simulink model "Observer_Controller_Sensors_P3"  (R2022a)
settings: Solver=ode45  StartTime=0.0  StopTime=20  RelTol=1e-3
values from neighbouring files (symbols this model uses):
  A = [0 0 1 0 0 ... (first row only)    [DesignProjectP2.m]    (also in DesignProjectP3.m; DesignProject_OffsetP3.m; mpc_example_regulation.m = [ 	 0,       0,              1,  0, 0; 	 0,       0,        ; mpc_example_tracking.m = [ 	 0,       0,              1,  0, 0; 	 0,       0,        )
  absolute_encoder_counts_per_revolution = 128    [ELEN90064_Project_Parameters.m]
  B = [0;0;0;0;1/La]    [DesignProjectP2.m]    (also in DesignProjectP3.m; DesignProject_OffsetP3.m; mpc_example_regulation.m = [0; 0; 0; 0; 1/La]; mpc_example_tracking.m = [0; 0; 0; 0; 1/La])
  C = [0 1 0 0 0]    [DesignProjectP2.m]    (also in DesignProjectP3.m = [1 0 0 0 0; DesignProject_OffsetP3.m = [1 0 0 0 0; mpc_example_regulation.m = [1 0 0 0 0; mpc_example_tracking.m = [1 0 0 0 0)
  Dp = c2d(Gp, T, 'zoh')    [DesignProjectP3.m]    (also in DesignProject_OffsetP3.m; mpc_example_regulation.m; mpc_example_tracking.m)
  gyro_sigma_drift = deg2rad(5)    [ELEN90064_Project_Parameters.m]
  init = [theta_m_init; theta_l_init; thetadot_m_init; thetadot_l_init; Ia_init]    [ELEN90064_Project_Parameters.m]
  K = K(2:6)    [DesignProjectP2.m]    (also in DesignProjectP3.m = Kr(2:6); DesignProject_OffsetP3.m = K_dist(2:6); phase2_emc.m = place(A,B,desired_poles))
  K_disc = Kr_disc(2:6)    [DesignProjectP3.m]    (also in DesignProject_OffsetP3.m)
  Ki = K(1:2)    [DesignProjectP2.m]    (also in DesignProjectP3.m = Kr(1); DesignProject_OffsetP3.m = K_dist(1))
  Ki_disc = Kr_disc(1)    [DesignProjectP3.m]    (also in DesignProject_OffsetP3.m)
  L = L_t'    [DesignProjectP3.m]    (also in DesignProject_OffsetP3.m; phase2_emc.m = place(A',C',desired_obsv_poles)')
  L_disc = L_disct'    [DesignProjectP3.m]    (also in DesignProject_OffsetP3.m; mpc_example_regulation.m; mpc_example_tracking.m)
  T = 1/50    (= 0.02)    [DesignProjectP3.m]    (also in DesignProject_OffsetP3.m; mpc_example_regulation.m; mpc_example_tracking.m)
  theta_l_init = deg2rad(0)    [ELEN90064_Project_Parameters.m]    (also in mpc_example_regulation.m; mpc_example_tracking.m)
  vision_fps = 50    [ELEN90064_Project_Parameters.m]
settings Model: Creator=Admin  LastModifiedBy=Admin

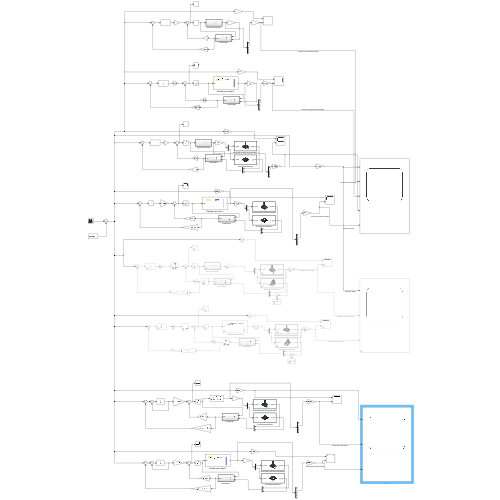
[thumbnail: Simulink's stored preview of the top-level diagram]
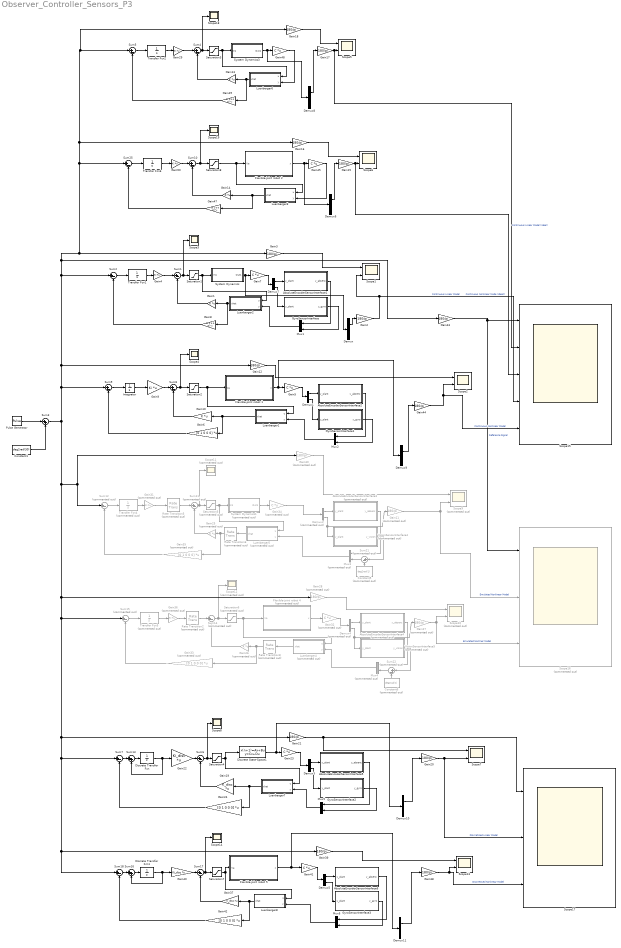
== system Observer_Controller_Sensors_P3 ==
  AbsoluteEncoderSensorInterface1 : Subsystem  TreatAsAtomicUnit=on
      mask Display: image('$imagefile'); % Use "Edit Image" on toolstrip to change.
  AbsoluteEncoderSensorInterface2 : Subsystem  TreatAsAtomicUnit=on
      mask Display: image('$imagefile'); % Use "Edit Image" on toolstrip to change.
  AbsoluteEncoderSensorInterface3 : Subsystem  Commented=on  TreatAsAtomicUnit=on
      mask Display: image('$imagefile'); % Use "Edit Image" on toolstrip to change.
  AbsoluteEncoderSensorInterface4 : Subsystem  Commented=on  TreatAsAtomicUnit=on
      mask Display: image('$imagefile'); % Use "Edit Image" on toolstrip to change.
  AbsoluteEncoderSensorInterface5 : Subsystem  TreatAsAtomicUnit=on
      mask Display: image('$imagefile'); % Use "Edit Image" on toolstrip to change.
  AbsoluteEncoderSensorInterface6 : Subsystem  TreatAsAtomicUnit=on
      mask Display: image('$imagefile'); % Use "Edit Image" on toolstrip to change.
  Constant1 : Constant  Value=deg2rad(30)
  Constant5 : Constant  Commented=on  Value=deg2rad(1)
  Constant6 : Constant  Commented=on  Value=deg2rad(1)
  Demux{,6,8..11} (6 alike) : Demux  Outputs=5
  Demux{1,3,5,7} (4 alike) : Demux  Outputs=2
  Demux2 : Demux  Commented=on  Outputs=2
  Demux4 : Demux  Commented=on  Outputs=2
  Discrete Transfer Fcn : DiscreteTransferFcn  Denominator=[1 0]
  Discrete Transfer Fcn1 : DiscreteTransferFcn  Denominator=[1 0]
  Discrete State-Space1 : DiscreteStateSpace  A=Dp.a  B=Dp.b  C=Dp.c  D=Dp.d  SampleTime=T
  Flexible-joint robot 1 : Subsystem
      mask Display: image('$imagefile'); % Use "Edit Image" on toolstrip to change.
  Flexible-joint robot 2 : Subsystem
      mask Display: image('$imagefile'); % Use "Edit Image" on toolstrip to change.
  Flexible-joint robot 4 : Subsystem  Commented=on
      mask Display: image('$imagefile'); % Use "Edit Image" on toolstrip to change.
  Flexible-joint robot 5 : Subsystem
      mask Display: image('$imagefile'); % Use "Edit Image" on toolstrip to change.
  Gain{1,10,13..14} (4 alike) : Gain  Gain=K  Multiplication=Matrix(K*u)
  Gain{11,27..28,30} (4 alike) : Gain  Commented=on  Gain=180/pi
  Gain{2..3,12,15..18,20..21,38..39,43..44} (13 alike) : Gain  Gain=180/pi
  Gain19 : Gain  Gain=K_disc  Multiplication=Matrix(K*u)
  Gain22 : Gain  Gain=Ki_disc  Multiplication=Matrix(K*u) (u vector)
  Gain{7,23,41,45,48} (5 alike) : Gain  Gain=C  Multiplication=Matrix(K*u)
  Gain{6,8,24,42,47,49} (6 alike) : Gain  Gain=[0 1 0 0 0]  Multiplication=Matrix(K*u)
  Gain25 : Gain  Commented=on  Gain=K  Multiplication=Matrix(K*u)
  Gain26 : Gain  Commented=on  Gain=K  Multiplication=Matrix(K*u)
  Gain29 : Gain  Gain=Ki  Multiplication=Matrix(K*u)
  Gain31 : Gain  Commented=on  Gain=Ki  Multiplication=Matrix(K*u)
  Gain32 : Gain  Commented=on  Gain=C  Multiplication=Matrix(K*u)
  Gain33 : Gain  Commented=on  Gain=[0 1 0 0 0]  Multiplication=Matrix(K*u)
  Gain34 : Gain  Commented=on  Gain=C  Multiplication=Matrix(K*u)
  Gain35 : Gain  Commented=on  Gain=[0 1 0 0 0]  Multiplication=Matrix(K*u)
  Gain36 : Gain  Commented=on  Gain=Ki  Multiplication=Matrix(K*u)
  Gain37 : Gain  Gain=K_disc  Multiplication=Matrix(K*u)
  Gain4 : Gain  Gain=Ki  Multiplication=Matrix(K*u)
  Gain40 : Gain  Gain=Ki_disc  Multiplication=Matrix(K*u)
  Gain5 : Gain  Gain=C  Multiplication=Matrix(K*u) (u vector)
  Gain50 : Gain  Gain=Ki  Multiplication=Matrix(K*u)
  Gain9 : Gain  Gain=Ki  Multiplication=Matrix(K*u) (u vector)
  GyroSensorInterface : Subsystem  TreatAsAtomicUnit=on
      mask Display: image('$imagefile'); % Use "Edit Image" on toolstrip to change.
  GyroSensorInterface1 : Subsystem  TreatAsAtomicUnit=on
      mask Display: image('$imagefile'); % Use "Edit Image" on toolstrip to change.
  GyroSensorInterface2 : Subsystem  TreatAsAtomicUnit=on
      mask Display: image('$imagefile'); % Use "Edit Image" on toolstrip to change.
  GyroSensorInterface3 : Subsystem  TreatAsAtomicUnit=on
      mask Display: image('$imagefile'); % Use "Edit Image" on toolstrip to change.
  Integrator : Integrator
  Luenberger1 : Subsystem  TreatAsAtomicUnit=on
  Luenberger2 : Subsystem  TreatAsAtomicUnit=on
  Luenberger3 : Subsystem  TreatAsAtomicUnit=on
  Luenberger4 : Subsystem  Commented=on  TreatAsAtomicUnit=on
  Luenberger5 : Subsystem  Commented=on  TreatAsAtomicUnit=on
  Luenberger6 : Subsystem  TreatAsAtomicUnit=on
  Luenberger7 : Subsystem  TreatAsAtomicUnit=on
  Luenberger8 : Subsystem  TreatAsAtomicUnit=on
  Mux{1..2,5..6} (4 alike) : Mux  Inputs=2
  Mux3 : Mux  Commented=on  Inputs=2
  Mux4 : Mux  Commented=on  Inputs=2
  Pulse Generator : DiscretePulseGenerator  PulseType=Time based  Amplitude=deg2rad(30)  Period=5  PulseWidth=50
  Rate Transition{2,5..6,8} (4 alike) : RateTransition  Commented=on  OutPortSampleTime=T
  Saturation{1..4,7..8} (6 alike) : Saturate  UpperLimit=6  LowerLimit=-6
  Saturation5 : Saturate  Commented=on  UpperLimit=6  LowerLimit=-6
  Saturation6 : Saturate  Commented=on  UpperLimit=6  LowerLimit=-6
  Scope{1..2,5..7,13} (6 alike) : Scope  NumInputPorts=2
  Scope10 : Scope  Commented=on  NumInputPorts=2
  Scope11 : Scope  Commented=on
  Scope12 : Scope  Commented=on
  Scope{3..4,8,14,18..19} (6 alike) : Scope
  Scope15 : Scope  NumInputPorts=5
  Scope16 : Scope  Commented=on  NumInputPorts=3
  Scope17 : Scope  NumInputPorts=3
  Scope9 : Scope  Commented=on  NumInputPorts=2
  Sum{1..2,4..10,17..18,25} (12 alike) : Sum  Inputs=|+-
  Sum{11..12,14..15,21..22} (6 alike) : Sum  Commented=on  Inputs=|+-
  Sum13 : Sum  Inputs=|++
  Sum16 : Sum  Inputs=|++
  Sum3 : Sum  Inputs=|++
  System Dynamics : Subsystem  TreatAsAtomicUnit=on
  System Dynamics1 : Subsystem  Commented=on  TreatAsAtomicUnit=on
  System Dynamics3 : Subsystem  TreatAsAtomicUnit=on
  Transfer Fcn1 : TransferFcn  Denominator=[1 0]
  Transfer Fcn2 : TransferFcn  Denominator=[1 0]
  Transfer Fcn4 : TransferFcn  Commented=on  Denominator=[1 0]
  Transfer Fcn5 : TransferFcn  Commented=on  Denominator=[1 0]
  Transfer Fcn6 : TransferFcn  Denominator=[1 0]
  VisionSensorInterface4 : Subsystem  Commented=on  TreatAsAtomicUnit=on
      mask Display: image('$imagefile'); % Use "Edit Image" on toolstrip to change.
  VisionSensorInterface5 : Subsystem  Commented=on  TreatAsAtomicUnit=on
      mask Display: image('$imagefile'); % Use "Edit Image" on toolstrip to change.
  wires:
  Sum8/1 -> Scope4/1, Saturation2/1
  Saturation2/1 -> Luenberger1/1(u), Flexible-joint robot 1/1(Va)
  Sum9/1 -> Integrator/1
  Gain10/1 -> Sum8/2
  Integrator/1 -> Gain9/1
  Flexible-joint robot 1/1(x) -> Demux9/1, Gain5/1
  Gain12/1 -> Scope2/1
  Gain44/1 -> Scope2/2, Scope15/5  "Continuous Nonlinear Model"
  Luenberger1/1(xhat) -> Gain6/1, Gain10/1
  Gain6/1 -> Sum9/2
  Gain9/1 -> Sum8/1
  Gain2/1 -> Scope1/2, Scope15/4  "Continuous Linear Model"
  Gain3/1 -> Scope1/1
  Transfer Fcn1/1 -> Gain4/1
  Gain1/1 -> Sum1/2
  Sum2/1 -> Transfer Fcn1/1
  Sum1/1 -> Scope3/1, Saturation1/1
  Gain8/1 -> Sum2/2
  Gain4/1 -> Sum1/1
  Saturation1/1 -> Luenberger2/1(u), System Dynamics/1(In1)
  Luenberger2/1(xhat) -> Gain8/1, Gain1/1
  Pulse Generator/1 -> Sum3/1
  System Dynamics/1(Out1) -> Demux/1, Gain7/1
  Constant1/1 -> Sum3/2
  Luenberger7/1(xhat) -> Gain24/1, Gain19/1
  Saturation4/1 -> Luenberger7/1(u), Discrete State-Space1/1
  Gain22/1 -> Sum6/1
  Gain24/1 -> Sum7/2
  Sum6/1 -> Saturation4/1, Scope8/1
  Gain19/1 -> Sum6/2
  Gain21/1 -> Scope17/1, Scope7/1
  Gain20/1 -> Scope17/2, Scope7/2  "Discretised Linear Model"
  Sum13/1 -> Discrete Transfer Fcn/1
  Discrete Transfer Fcn/1 -> Gain22/1, Sum13/2
  Sum7/1 -> Sum13/1
  Gain23/1 -> Demux3/1
  System Dynamics1/1(Out1) -> Gain34/1
  Luenberger5/1(xhat) -> Rate Transition6/1
  Saturation5/1 -> System Dynamics1/1(In1), Luenberger5/1(u)
  Gain31/1 -> Rate Transition5/1
  Gain35/1 -> Sum12/2
  Sum11/1 -> Saturation5/1, Scope11/1
  Sum12/1 -> Transfer Fcn4/1
  Gain25/1 -> Sum11/2
  Transfer Fcn4/1 -> Gain31/1
  Gain30/1 -> Scope9/1
  Gain36/1 -> Rate Transition2/1
  Gain33/1 -> Sum15/2
  Luenberger4/1(xhat) -> Rate Transition8/1
  Gain32/1 -> Demux4/1
  Gain27/1 -> Scope10/2, Scope16/3  "Emulated Nonliner Model"
  Gain28/1 -> Scope10/1
  Flexible-joint robot 4/1(x) -> Gain32/1
  Transfer Fcn5/1 -> Gain36/1
  Sum15/1 -> Transfer Fcn5/1
  Saturation6/1 -> Flexible-joint robot 4/1(Va), Luenberger4/1(u)
  Sum14/1 -> Saturation6/1, Scope12/1
  Gain26/1 -> Sum14/2
  Rate Transition2/1 -> Sum14/1
  Gain41/1 -> Demux5/1
  Sum18/1 -> Sum16/1
  Discrete Transfer Fcn1/1 -> Sum16/2, Gain40/1
  Sum16/1 -> Discrete Transfer Fcn1/1
  Gain38/1 -> Scope13/2, Scope17/3  "Discretised Nonlinear Model"
  Gain39/1 -> Scope13/1
  Gain37/1 -> Sum17/2
  Sum17/1 -> Scope14/1, Saturation7/1
  Gain42/1 -> Sum18/2
  Gain40/1 -> Sum17/1
  Saturation7/1 -> Flexible-joint robot 5/1(Va), Luenberger8/1(u)
  Luenberger8/1(xhat) -> Gain37/1, Gain42/1
  Rate Transition5/1 -> Sum11/1
  Rate Transition6/1 -> Gain35/1, Gain25/1
  Gain43/1 -> Scope16/1, Scope15/1  "Reference Signal"
  Rate Transition8/1 -> Gain33/1, Gain26/1
  GyroSensorInterface/1(y_gyro) -> Mux1/2
  AbsoluteEncoderSensorInterface1/1(y_absenc) -> Mux1/1
  Gain7/1 -> Demux7/1
  Demux7/2 -> GyroSensorInterface/1(y_plant)
  Demux7/1 -> AbsoluteEncoderSensorInterface1/1(y_plant)
  Mux1/1 -> Luenberger2/2(y)
  Mux2/1 -> Luenberger1/2(y)
  Demux1/1 -> AbsoluteEncoderSensorInterface2/1(y_plant)
  Demux1/2 -> GyroSensorInterface1/1(y_plant)
  Gain5/1 -> Demux1/1
  AbsoluteEncoderSensorInterface2/1(y_absenc) -> Mux2/1
  GyroSensorInterface1/1(y_gyro) -> Mux2/2
  VisionSensorInterface4/1(y_vision) -> Sum21/1
  Constant5/1 -> Sum21/2
  Sum21/1 -> Mux3/2
  AbsoluteEncoderSensorInterface3/1(y_absenc) -> Mux3/1
  Demux2/2 -> Gain11/1, VisionSensorInterface4/1(y_plant)
  Demux2/1 -> AbsoluteEncoderSensorInterface3/1(y_plant)
  Mux3/1 -> Luenberger5/2(y)
  Gain34/1 -> Demux2/1
  Gain11/1 -> Scope9/2, Scope16/2  "Emulated Nonlinear Model"
  Mux4/1 -> Luenberger4/2(y)
  Demux4/1 -> AbsoluteEncoderSensorInterface4/1(y_plant)
  Demux4/2 -> VisionSensorInterface5/1(y_plant), Gain27/1
  AbsoluteEncoderSensorInterface4/1(y_absenc) -> Mux4/1
  Sum22/1 -> Mux4/2
  Constant6/1 -> Sum22/2
  VisionSensorInterface5/1(y_vision) -> Sum22/1
  AbsoluteEncoderSensorInterface5/1(y_absenc) -> Mux5/1
  Demux3/1 -> AbsoluteEncoderSensorInterface5/1(y_plant)
  Demux3/2 -> GyroSensorInterface2/1(y_plant)
  Demux5/2 -> GyroSensorInterface3/1(y_plant)
  Demux5/1 -> AbsoluteEncoderSensorInterface6/1(y_plant)
  AbsoluteEncoderSensorInterface6/1(y_absenc) -> Mux6/1
  GyroSensorInterface3/1(y_gyro) -> Mux6/2
  Gain18/1 -> Scope5/1
  Transfer Fcn6/1 -> Gain50/1
  Sum4/1 -> Scope18/1, Saturation3/1
  Sum25/1 -> Transfer Fcn6/1
  Gain48/1 -> Luenberger6/2(y)
  Saturation3/1 -> Luenberger6/1(u), System Dynamics3/1(In1)
  Gain29/1 -> Sum4/1
  Gain14/1 -> Sum10/2
  Transfer Fcn2/1 -> Gain29/1
  Gain17/1 -> Scope15/2, Scope5/2  "Continuous Linear Model (Ideal)"
  System Dynamics3/1(Out1) -> Demux8/1, Gain48/1
  Gain13/1 -> Sum4/2
  Luenberger6/1(xhat) -> Gain49/1, Gain13/1
  Gain49/1 -> Sum5/2
  Gain47/1 -> Sum25/2
  Gain50/1 -> Sum10/1
  Saturation8/1 -> Luenberger3/1(u), Flexible-joint robot 2/1(Va)
  Gain15/1 -> Scope15/3, Scope6/2  "Continuous Nonlinear Mode (Ideal)l"
  Sum10/1 -> Scope19/1, Saturation8/1
  Demux8/2 -> Gain17/1
  Sum5/1 -> Transfer Fcn2/1
  Gain16/1 -> Scope6/1
  Sum3/1 -> Gain12/1, Gain18/1, Sum5/1, Gain16/1, Sum25/1, Gain3/1, Gain43/1, Sum2/1, Sum9/1, Sum12/1, Gain30/1, Gain28/1, Gain21/1, Sum18/1, Gain39/1, Sum7/1, Sum15/1
  Discrete State-Space1/1 -> Demux10/1, Gain23/1
  Flexible-joint robot 5/1(x) -> Demux11/1, Gain41/1
  GyroSensorInterface2/1(y_gyro) -> Mux5/2
  Demux6/2 -> Gain15/1
  Demux/2 -> Gain2/1
  Demux9/2 -> Gain44/1
  Flexible-joint robot 2/1(x) -> Demux6/1, Gain45/1
  Gain45/1 -> Luenberger3/2(y)
  Luenberger3/1(xhat) -> Gain47/1, Gain14/1
  Mux5/1 -> Luenberger7/2(y)
  Demux10/2 -> Gain20/1
  Demux11/2 -> Gain38/1
  Mux6/1 -> Luenberger8/2(y)

== system Observer_Controller_Sensors_P3/AbsoluteEncoderSensorInterface1 ==
  note: Notes:
      | > This sensor block is protected.
      | > The AbsoluteEncoderSensor.slxp file needs to be on the Matlab path in order to simulate this sensor.
      | > You should have download the .slpx file appropriate for you operating system {Windows, Mac, Linux}.
      | > The constant parameters on the left are set in the " ELEN90064_Project_Parameters.m " script.
      | > The sensors appendix in project description provides a 1-page summary of the sensor model and of how each parameters relates to the expected performance of the sensor.
      | > You should read the relevant page of that appendix before using this sensor.
  y_plant : Inport
  AbsoluteEncoderSensor : ModelReference  ModelNameDialog=AbsoluteEncoderSensor.slxp  ModelReferenceVersion=1.16  CopyOfModelProtected=on
  NUMBER OF COUNTS PER REVOLUTION : Constant  Value=absolute_encoder_counts_per_revolution
  y_absenc : Outport
  wires:
  NUMBER OF COUNTS PER REVOLUTION/1 -> AbsoluteEncoderSensor/1
  y_plant/1 -> AbsoluteEncoderSensor/2
  AbsoluteEncoderSensor/1 -> y_absenc/1

== system Observer_Controller_Sensors_P3/AbsoluteEncoderSensorInterface2 ==
  note: Notes:
      | > This sensor block is protected.
      | > The AbsoluteEncoderSensor.slxp file needs to be on the Matlab path in order to simulate this sensor.
      | > You should have download the .slpx file appropriate for you operating system {Windows, Mac, Linux}.
      | > The constant parameters on the left are set in the " ELEN90064_Project_Parameters.m " script.
      | > The sensors appendix in project description provides a 1-page summary of the sensor model and of how each parameters relates to the expected performance of the sensor.
      | > You should read the relevant page of that appendix before using this sensor.
  y_plant : Inport
  AbsoluteEncoderSensor : ModelReference  ModelNameDialog=AbsoluteEncoderSensor.slxp  ModelReferenceVersion=1.16  CopyOfModelProtected=on
  NUMBER OF COUNTS PER REVOLUTION : Constant  Value=absolute_encoder_counts_per_revolution
  y_absenc : Outport
  wires:
  AbsoluteEncoderSensor/1 -> y_absenc/1
  y_plant/1 -> AbsoluteEncoderSensor/2
  NUMBER OF COUNTS PER REVOLUTION/1 -> AbsoluteEncoderSensor/1

== system Observer_Controller_Sensors_P3/AbsoluteEncoderSensorInterface3 ==
  note: Notes:
      | > This sensor block is protected.
      | > The AbsoluteEncoderSensor.slxp file needs to be on the Matlab path in order to simulate this sensor.
      | > You should have download the .slpx file appropriate for you operating system {Windows, Mac, Linux}.
      | > The constant parameters on the left are set in the " ELEN90064_Project_Parameters.m " script.
      | > The sensors appendix in project description provides a 1-page summary of the sensor model and of how each parameters relates to the expected performance of the sensor.
      | > You should read the relevant page of that appendix before using this sensor.
  y_plant : Inport
  AbsoluteEncoderSensor : ModelReference  ModelNameDialog=AbsoluteEncoderSensor.slxp  ModelReferenceVersion=1.16  CopyOfModelProtected=on
  NUMBER OF COUNTS PER REVOLUTION : Constant  Value=absolute_encoder_counts_per_revolution
  y_absenc : Outport
  wires:
  NUMBER OF COUNTS PER REVOLUTION/1 -> AbsoluteEncoderSensor/1
  y_plant/1 -> AbsoluteEncoderSensor/2
  AbsoluteEncoderSensor/1 -> y_absenc/1

== system Observer_Controller_Sensors_P3/AbsoluteEncoderSensorInterface4 ==
  note: Notes:
      | > This sensor block is protected.
      | > The AbsoluteEncoderSensor.slxp file needs to be on the Matlab path in order to simulate this sensor.
      | > You should have download the .slpx file appropriate for you operating system {Windows, Mac, Linux}.
      | > The constant parameters on the left are set in the " ELEN90064_Project_Parameters.m " script.
      | > The sensors appendix in project description provides a 1-page summary of the sensor model and of how each parameters relates to the expected performance of the sensor.
      | > You should read the relevant page of that appendix before using this sensor.
  y_plant : Inport
  AbsoluteEncoderSensor : ModelReference  ModelNameDialog=AbsoluteEncoderSensor.slxp  ModelReferenceVersion=1.16  CopyOfModelProtected=on
  NUMBER OF COUNTS PER REVOLUTION : Constant  Value=absolute_encoder_counts_per_revolution
  y_absenc : Outport
  wires:
  AbsoluteEncoderSensor/1 -> y_absenc/1
  y_plant/1 -> AbsoluteEncoderSensor/2
  NUMBER OF COUNTS PER REVOLUTION/1 -> AbsoluteEncoderSensor/1

== system Observer_Controller_Sensors_P3/AbsoluteEncoderSensorInterface5 ==
  note: Notes:
      | > This sensor block is protected.
      | > The AbsoluteEncoderSensor.slxp file needs to be on the Matlab path in order to simulate this sensor.
      | > You should have download the .slpx file appropriate for you operating system {Windows, Mac, Linux}.
      | > The constant parameters on the left are set in the " ELEN90064_Project_Parameters.m " script.
      | > The sensors appendix in project description provides a 1-page summary of the sensor model and of how each parameters relates to the expected performance of the sensor.
      | > You should read the relevant page of that appendix before using this sensor.
  y_plant : Inport
  AbsoluteEncoderSensor : ModelReference  ModelNameDialog=AbsoluteEncoderSensor.slxp  ModelReferenceVersion=1.16  CopyOfModelProtected=on
  NUMBER OF COUNTS PER REVOLUTION : Constant  Value=absolute_encoder_counts_per_revolution
  y_absenc : Outport
  wires:
  NUMBER OF COUNTS PER REVOLUTION/1 -> AbsoluteEncoderSensor/1
  y_plant/1 -> AbsoluteEncoderSensor/2
  AbsoluteEncoderSensor/1 -> y_absenc/1

== system Observer_Controller_Sensors_P3/AbsoluteEncoderSensorInterface6 ==
  note: Notes:
      | > This sensor block is protected.
      | > The AbsoluteEncoderSensor.slxp file needs to be on the Matlab path in order to simulate this sensor.
      | > You should have download the .slpx file appropriate for you operating system {Windows, Mac, Linux}.
      | > The constant parameters on the left are set in the " ELEN90064_Project_Parameters.m " script.
      | > The sensors appendix in project description provides a 1-page summary of the sensor model and of how each parameters relates to the expected performance of the sensor.
      | > You should read the relevant page of that appendix before using this sensor.
  y_plant : Inport
  AbsoluteEncoderSensor : ModelReference  ModelNameDialog=AbsoluteEncoderSensor.slxp  ModelReferenceVersion=1.16  CopyOfModelProtected=on
  NUMBER OF COUNTS PER REVOLUTION : Constant  Value=absolute_encoder_counts_per_revolution
  y_absenc : Outport
  wires:
  AbsoluteEncoderSensor/1 -> y_absenc/1
  y_plant/1 -> AbsoluteEncoderSensor/2
  NUMBER OF COUNTS PER REVOLUTION/1 -> AbsoluteEncoderSensor/1

== system Observer_Controller_Sensors_P3/Flexible-joint robot 1 ==
  Va : Inport
  Constant : Constant  Value=init
  Constant1 : Constant  Value=0
  Flexible-joint robot 1 : ModelReference  ModelNameDialog=Flexible_joint_robot_1  ModelReferenceVersion=1.65  CopyOfModelProtected=on
  Step : Step  After=0.05  SampleTime=0
  x : Outport
  wires:
  Constant/1 -> Flexible-joint robot 1/2
  Constant1/1 -> Flexible-joint robot 1/3
  Flexible-joint robot 1/1 -> x/1
  Va/1 -> Flexible-joint robot 1/1

== system Observer_Controller_Sensors_P3/Flexible-joint robot 2 ==
  Va : Inport
  Constant : Constant  Value=init
  Constant1 : Constant  Value=0
  Flexible-joint robot 1 : ModelReference  ModelNameDialog=Flexible_joint_robot_1  ModelReferenceVersion=1.65  CopyOfModelProtected=on
  Step : Step  After=0.05  SampleTime=0
  x : Outport
  wires:
  Constant/1 -> Flexible-joint robot 1/2
  Constant1/1 -> Flexible-joint robot 1/3
  Flexible-joint robot 1/1 -> x/1
  Va/1 -> Flexible-joint robot 1/1

== system Observer_Controller_Sensors_P3/Flexible-joint robot 4 ==
  Va : Inport
  Constant : Constant  Value=init
  Constant1 : Constant  Value=0
  Flexible-joint robot 1 : ModelReference  ModelNameDialog=Flexible_joint_robot_1  ModelReferenceVersion=1.65  CopyOfModelProtected=on
  Step : Step  After=0.05  SampleTime=0
  x : Outport
  wires:
  Va/1 -> Flexible-joint robot 1/1
  Flexible-joint robot 1/1 -> x/1
  Constant1/1 -> Flexible-joint robot 1/3
  Constant/1 -> Flexible-joint robot 1/2

== system Observer_Controller_Sensors_P3/Flexible-joint robot 5 ==
  Va : Inport
  Constant : Constant  Value=init
  Constant1 : Constant  Value=0
  Flexible-joint robot 1 : ModelReference  ModelNameDialog=Flexible_joint_robot_1  ModelReferenceVersion=1.65  CopyOfModelProtected=on
  Step : Step  After=0.05  SampleTime=0
  x : Outport
  wires:
  Constant/1 -> Flexible-joint robot 1/2
  Constant1/1 -> Flexible-joint robot 1/3
  Flexible-joint robot 1/1 -> x/1
  Va/1 -> Flexible-joint robot 1/1

== system Observer_Controller_Sensors_P3/GyroSensorInterface ==
  note: Notes:
      | > This sensor block is protected.
      | > The GyroSensor.slxp file needs to be on the Matlab path in order to simulate this sensor.
      | > You should have download the .slpx file appropriate for you operating system {Windows, Mac, Linux}.
      | > The constant parameters on the left are set in the " ELEN90064_Project_Parameters.m " script.
      | > The sensors appendix in project description provides a 1-page summary of the sensor model and of how each parameters relates to the expected performance of the sensor.
      | > You should read the relevant page of that appendix before using this sensor.
  y_plant : Inport
  GYRO SIGMA DRIFT [rad/s^2] : Constant  Value=gyro_sigma_drift
  GyroSensor : ModelReference  ModelNameDialog=GyroSensor.slxp  ModelReferenceVersion=1.18  CopyOfModelProtected=on
  y_gyro : Outport
  wires:
  GYRO SIGMA DRIFT [rad/s^2]/1 -> GyroSensor/1
  y_plant/1 -> GyroSensor/2
  GyroSensor/1 -> y_gyro/1

== system Observer_Controller_Sensors_P3/GyroSensorInterface1 ==
  note: Notes:
      | > This sensor block is protected.
      | > The GyroSensor.slxp file needs to be on the Matlab path in order to simulate this sensor.
      | > You should have download the .slpx file appropriate for you operating system {Windows, Mac, Linux}.
      | > The constant parameters on the left are set in the " ELEN90064_Project_Parameters.m " script.
      | > The sensors appendix in project description provides a 1-page summary of the sensor model and of how each parameters relates to the expected performance of the sensor.
      | > You should read the relevant page of that appendix before using this sensor.
  y_plant : Inport
  GYRO SIGMA DRIFT [rad/s^2] : Constant  Value=gyro_sigma_drift
  GyroSensor : ModelReference  ModelNameDialog=GyroSensor.slxp  ModelReferenceVersion=1.18  CopyOfModelProtected=on
  y_gyro : Outport
  wires:
  GYRO SIGMA DRIFT [rad/s^2]/1 -> GyroSensor/1
  y_plant/1 -> GyroSensor/2
  GyroSensor/1 -> y_gyro/1

== system Observer_Controller_Sensors_P3/GyroSensorInterface2 ==
  note: Notes:
      | > This sensor block is protected.
      | > The GyroSensor.slxp file needs to be on the Matlab path in order to simulate this sensor.
      | > You should have download the .slpx file appropriate for you operating system {Windows, Mac, Linux}.
      | > The constant parameters on the left are set in the " ELEN90064_Project_Parameters.m " script.
      | > The sensors appendix in project description provides a 1-page summary of the sensor model and of how each parameters relates to the expected performance of the sensor.
      | > You should read the relevant page of that appendix before using this sensor.
  y_plant : Inport
  GYRO SIGMA DRIFT [rad/s^2] : Constant  Value=gyro_sigma_drift
  GyroSensor : ModelReference  ModelNameDialog=GyroSensor.slxp  ModelReferenceVersion=1.18  CopyOfModelProtected=on
  y_gyro : Outport
  wires:
  GYRO SIGMA DRIFT [rad/s^2]/1 -> GyroSensor/1
  y_plant/1 -> GyroSensor/2
  GyroSensor/1 -> y_gyro/1

== system Observer_Controller_Sensors_P3/GyroSensorInterface3 ==
  note: Notes:
      | > This sensor block is protected.
      | > The GyroSensor.slxp file needs to be on the Matlab path in order to simulate this sensor.
      | > You should have download the .slpx file appropriate for you operating system {Windows, Mac, Linux}.
      | > The constant parameters on the left are set in the " ELEN90064_Project_Parameters.m " script.
      | > The sensors appendix in project description provides a 1-page summary of the sensor model and of how each parameters relates to the expected performance of the sensor.
      | > You should read the relevant page of that appendix before using this sensor.
  y_plant : Inport
  GYRO SIGMA DRIFT [rad/s^2] : Constant  Value=gyro_sigma_drift
  GyroSensor : ModelReference  ModelNameDialog=GyroSensor.slxp  ModelReferenceVersion=1.18  CopyOfModelProtected=on
  y_gyro : Outport
  wires:
  GYRO SIGMA DRIFT [rad/s^2]/1 -> GyroSensor/1
  y_plant/1 -> GyroSensor/2
  GyroSensor/1 -> y_gyro/1

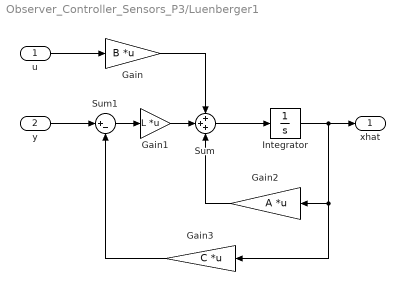
== system Observer_Controller_Sensors_P3/Luenberger1 ==
  u : Inport
  y : Inport  Port=2
  Gain : Gain  Gain=B  Multiplication=Matrix(K*u) (u vector)
  Gain1 : Gain  Gain=L  Multiplication=Matrix(K*u) (u vector)
  Gain2 : Gain  Gain=A  Multiplication=Matrix(K*u) (u vector)
  Gain3 : Gain  Gain=C  Multiplication=Matrix(K*u) (u vector)
  Integrator : Integrator
  Sum : Sum  Inputs=+++
  Sum1 : Sum  Inputs=|+-
  xhat : Outport
  wires:
  u/1 -> Gain/1
  Gain/1 -> Sum/1
  y/1 -> Sum1/1
  Sum1/1 -> Gain1/1
  Gain1/1 -> Sum/2
  Sum/1 -> Integrator/1
  Integrator/1 -> Gain3/1, Gain2/1, xhat/1
  Gain2/1 -> Sum/3
  Gain3/1 -> Sum1/2

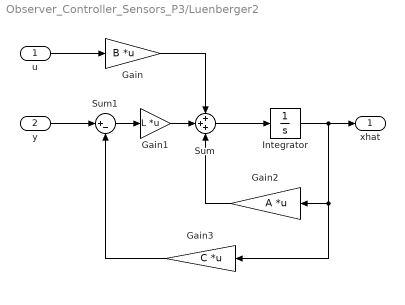
== system Observer_Controller_Sensors_P3/Luenberger2 ==
  u : Inport
  y : Inport  Port=2
  Gain : Gain  Gain=B  Multiplication=Matrix(K*u) (u vector)
  Gain1 : Gain  Gain=L  Multiplication=Matrix(K*u) (u vector)
  Gain2 : Gain  Gain=A  Multiplication=Matrix(K*u) (u vector)
  Gain3 : Gain  Gain=C  Multiplication=Matrix(K*u) (u vector)
  Integrator : Integrator
  Sum : Sum  Inputs=+++
  Sum1 : Sum  Inputs=|+-
  xhat : Outport
  wires:
  u/1 -> Gain/1
  Gain/1 -> Sum/1
  y/1 -> Sum1/1
  Sum1/1 -> Gain1/1
  Gain1/1 -> Sum/2
  Sum/1 -> Integrator/1
  Integrator/1 -> Gain3/1, Gain2/1, xhat/1
  Gain2/1 -> Sum/3
  Gain3/1 -> Sum1/2

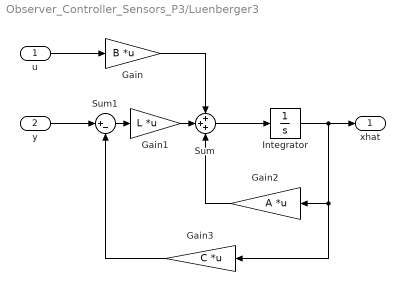
== system Observer_Controller_Sensors_P3/Luenberger3 ==
  u : Inport
  y : Inport  Port=2
  Gain : Gain  Gain=B  Multiplication=Matrix(K*u) (u vector)
  Gain1 : Gain  Gain=L  Multiplication=Matrix(K*u) (u vector)
  Gain2 : Gain  Gain=A  Multiplication=Matrix(K*u) (u vector)
  Gain3 : Gain  Gain=C  Multiplication=Matrix(K*u) (u vector)
  Integrator : Integrator
  Sum : Sum  Inputs=+++
  Sum1 : Sum  Inputs=|+-
  xhat : Outport
  wires:
  u/1 -> Gain/1
  Gain/1 -> Sum/1
  y/1 -> Sum1/1
  Sum1/1 -> Gain1/1
  Gain1/1 -> Sum/2
  Sum/1 -> Integrator/1
  Integrator/1 -> Gain3/1, Gain2/1, xhat/1
  Gain2/1 -> Sum/3
  Gain3/1 -> Sum1/2

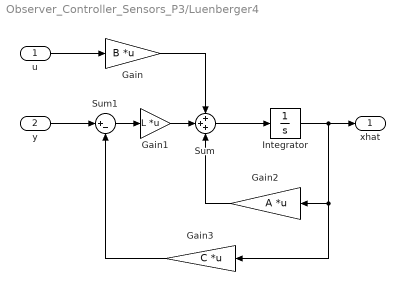
== system Observer_Controller_Sensors_P3/Luenberger4 ==
  u : Inport
  y : Inport  Port=2
  Gain : Gain  Gain=B  Multiplication=Matrix(K*u) (u vector)
  Gain1 : Gain  Gain=L  Multiplication=Matrix(K*u) (u vector)
  Gain2 : Gain  Gain=A  Multiplication=Matrix(K*u) (u vector)
  Gain3 : Gain  Gain=C  Multiplication=Matrix(K*u) (u vector)
  Integrator : Integrator
  Sum : Sum  Inputs=+++
  Sum1 : Sum  Inputs=|+-
  xhat : Outport
  wires:
  Gain3/1 -> Sum1/2
  Gain2/1 -> Sum/3
  Integrator/1 -> xhat/1, Gain2/1, Gain3/1
  Sum/1 -> Integrator/1
  Gain1/1 -> Sum/2
  Sum1/1 -> Gain1/1
  y/1 -> Sum1/1
  Gain/1 -> Sum/1
  u/1 -> Gain/1

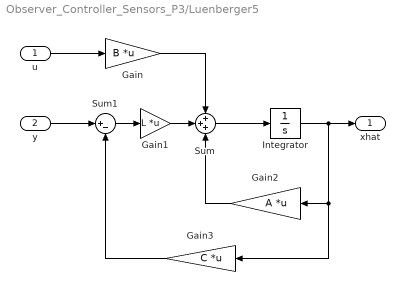
== system Observer_Controller_Sensors_P3/Luenberger5 ==
  u : Inport
  y : Inport  Port=2
  Gain : Gain  Gain=B  Multiplication=Matrix(K*u) (u vector)
  Gain1 : Gain  Gain=L  Multiplication=Matrix(K*u) (u vector)
  Gain2 : Gain  Gain=A  Multiplication=Matrix(K*u) (u vector)
  Gain3 : Gain  Gain=C  Multiplication=Matrix(K*u) (u vector)
  Integrator : Integrator
  Sum : Sum  Inputs=+++
  Sum1 : Sum  Inputs=|+-
  xhat : Outport
  wires:
  Gain3/1 -> Sum1/2
  Gain2/1 -> Sum/3
  Integrator/1 -> xhat/1, Gain2/1, Gain3/1
  Sum/1 -> Integrator/1
  Gain1/1 -> Sum/2
  Sum1/1 -> Gain1/1
  y/1 -> Sum1/1
  Gain/1 -> Sum/1
  u/1 -> Gain/1

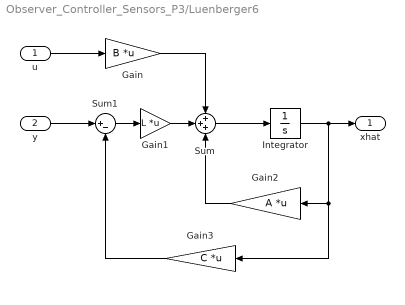
== system Observer_Controller_Sensors_P3/Luenberger6 ==
  u : Inport
  y : Inport  Port=2
  Gain : Gain  Gain=B  Multiplication=Matrix(K*u) (u vector)
  Gain1 : Gain  Gain=L  Multiplication=Matrix(K*u) (u vector)
  Gain2 : Gain  Gain=A  Multiplication=Matrix(K*u) (u vector)
  Gain3 : Gain  Gain=C  Multiplication=Matrix(K*u) (u vector)
  Integrator : Integrator
  Sum : Sum  Inputs=+++
  Sum1 : Sum  Inputs=|+-
  xhat : Outport
  wires:
  u/1 -> Gain/1
  Gain/1 -> Sum/1
  y/1 -> Sum1/1
  Sum1/1 -> Gain1/1
  Gain1/1 -> Sum/2
  Sum/1 -> Integrator/1
  Integrator/1 -> Gain3/1, Gain2/1, xhat/1
  Gain2/1 -> Sum/3
  Gain3/1 -> Sum1/2

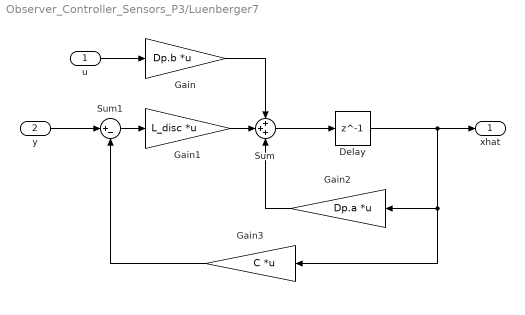
== system Observer_Controller_Sensors_P3/Luenberger7 ==
  u : Inport
  y : Inport  Port=2
  Delay : Delay  DelayLength=1
  Gain : Gain  Gain=Dp.b  Multiplication=Matrix(K*u) (u vector)
  Gain1 : Gain  Gain=L_disc  Multiplication=Matrix(K*u) (u vector)
  Gain2 : Gain  Gain=Dp.a  Multiplication=Matrix(K*u) (u vector)
  Gain3 : Gain  Gain=C  Multiplication=Matrix(K*u) (u vector)
  Sum : Sum  Inputs=+++
  Sum1 : Sum  Inputs=|+-
  xhat : Outport
  wires:
  u/1 -> Gain/1
  Gain/1 -> Sum/1
  y/1 -> Sum1/1
  Sum1/1 -> Gain1/1
  Gain1/1 -> Sum/2
  Sum/1 -> Delay/1
  Delay/1 -> Gain3/1, Gain2/1, xhat/1
  Gain2/1 -> Sum/3
  Gain3/1 -> Sum1/2

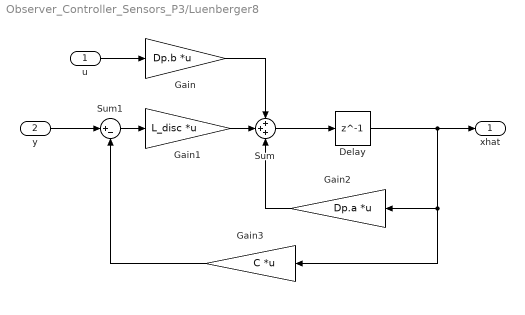
== system Observer_Controller_Sensors_P3/Luenberger8 ==
  u : Inport
  y : Inport  Port=2
  Delay : Delay  DelayLength=1
  Gain : Gain  Gain=Dp.b  Multiplication=Matrix(K*u) (u vector)
  Gain1 : Gain  Gain=L_disc  Multiplication=Matrix(K*u) (u vector)
  Gain2 : Gain  Gain=Dp.a  Multiplication=Matrix(K*u) (u vector)
  Gain3 : Gain  Gain=C  Multiplication=Matrix(K*u) (u vector)
  Sum : Sum  Inputs=+++
  Sum1 : Sum  Inputs=|+-
  xhat : Outport
  wires:
  u/1 -> Gain/1
  Gain/1 -> Sum/1
  y/1 -> Sum1/1
  Sum1/1 -> Gain1/1
  Gain1/1 -> Sum/2
  Sum/1 -> Delay/1
  Delay/1 -> Gain3/1, Gain2/1, xhat/1
  Gain2/1 -> Sum/3
  Gain3/1 -> Sum1/2

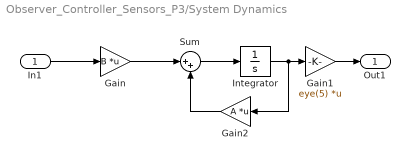
== system Observer_Controller_Sensors_P3/System Dynamics ==
  In1 : Inport
  Gain : Gain  Gain=B  Multiplication=Matrix(K*u)
  Gain1 : Gain  Gain=eye(5)  Multiplication=Matrix(K*u)
  Gain2 : Gain  Gain=A  Multiplication=Matrix(K*u)
  Integrator : Integrator
  Sum : Sum  Inputs=|++
  Out1 : Outport
  wires:
  In1/1 -> Gain/1
  Gain/1 -> Sum/1
  Sum/1 -> Integrator/1
  Integrator/1 -> Gain2/1, Gain1/1
  Gain1/1 -> Out1/1
  Gain2/1 -> Sum/2

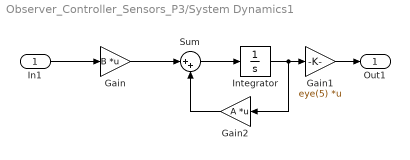
== system Observer_Controller_Sensors_P3/System Dynamics1 ==
  In1 : Inport
  Gain : Gain  Gain=B  Multiplication=Matrix(K*u)
  Gain1 : Gain  Gain=eye(5)  Multiplication=Matrix(K*u)
  Gain2 : Gain  Gain=A  Multiplication=Matrix(K*u)
  Integrator : Integrator
  Sum : Sum  Inputs=|++
  Out1 : Outport
  wires:
  Gain2/1 -> Sum/2
  Gain1/1 -> Out1/1
  Integrator/1 -> Gain1/1, Gain2/1
  Sum/1 -> Integrator/1
  Gain/1 -> Sum/1
  In1/1 -> Gain/1

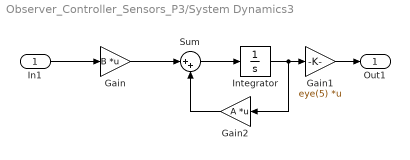
== system Observer_Controller_Sensors_P3/System Dynamics3 ==
  In1 : Inport
  Gain : Gain  Gain=B  Multiplication=Matrix(K*u)
  Gain1 : Gain  Gain=eye(5)  Multiplication=Matrix(K*u)
  Gain2 : Gain  Gain=A  Multiplication=Matrix(K*u)
  Integrator : Integrator
  Sum : Sum  Inputs=|++
  Out1 : Outport
  wires:
  In1/1 -> Gain/1
  Gain/1 -> Sum/1
  Sum/1 -> Integrator/1
  Integrator/1 -> Gain2/1, Gain1/1
  Gain1/1 -> Out1/1
  Gain2/1 -> Sum/2

== system Observer_Controller_Sensors_P3/VisionSensorInterface4 ==
  note: Notes:
      | > This sensor block is protected.
      | > The VisionSensor.slxp file needs to be on the Matlab path in order to simulate this sensor.
      | > You should have download the .slpx file appropriate for you operating system {Windows, Mac, Linux}.
      | > The constant parameters on the left are set in the "ELEN90064_Project_Parameters.m" script.
      | > The sensors appendix in project description provides a 1-page summary of the sensor model and of how each parameters relates to the expected performance of the sensor.
      | > You should read the relevant page of that appendix before using this sensor.
  y_plant : Inport
  INITIAL LINK ANGLE [rad] : Constant  Value=theta_l_init
  VISION FRAME RATE [fps] : Constant  Value=vision_fps
  VisionSensor : ModelReference  ModelNameDialog=VisionSensor.slxp  ModelReferenceVersion=1.19  CopyOfModelProtected=on
  y_vision : Outport
  wires:
  VisionSensor/1 -> y_vision/1
  y_plant/1 -> VisionSensor/3
  INITIAL LINK ANGLE [rad]/1 -> VisionSensor/2
  VISION FRAME RATE [fps]/1 -> VisionSensor/1

== system Observer_Controller_Sensors_P3/VisionSensorInterface5 ==
  note: Notes:
      | > This sensor block is protected.
      | > The VisionSensor.slxp file needs to be on the Matlab path in order to simulate this sensor.
      | > You should have download the .slpx file appropriate for you operating system {Windows, Mac, Linux}.
      | > The constant parameters on the left are set in the "ELEN90064_Project_Parameters.m" script.
      | > The sensors appendix in project description provides a 1-page summary of the sensor model and of how each parameters relates to the expected performance of the sensor.
      | > You should read the relevant page of that appendix before using this sensor.
  y_plant : Inport
  INITIAL LINK ANGLE [rad] : Constant  Value=theta_l_init
  VISION FRAME RATE [fps] : Constant  Value=vision_fps
  VisionSensor : ModelReference  ModelNameDialog=VisionSensor.slxp  ModelReferenceVersion=1.19  CopyOfModelProtected=on
  y_vision : Outport
  wires:
  VISION FRAME RATE [fps]/1 -> VisionSensor/1
  INITIAL LINK ANGLE [rad]/1 -> VisionSensor/2
  y_plant/1 -> VisionSensor/3
  VisionSensor/1 -> y_vision/1
